simulink model "test_com_SensorFusion_SF_E10_fuerE9Daten"  (R2019b)
settings: Solver=FixedStepDiscrete  StartTime=0  StopTime=85  FixedStep=0.001  RelTol=1e-3
undefined symbols (not defined in the file or in its folder): BxTM, ByTM, CxTM, CyTM, g, gamma_stat_front, gamma_stat_rear, gearbox_ratio, l_F, l_R, m_sprung, m_unsprung_quarter, mag_calib_front_center, mag_calib_front_compmatrix, mag_calib_rear_center, mag_calib_rear_compmatrix, param, switch_VelYcalculation_pSF, testStart_VelX_pSF, testVelY_pSF, tire_r_dyn, track_angle_front, track_width_front, track_width_rear, v2o_x, wheel_kinematics_breakpoints, wheel_kinematics_FL_data, wheel_kinematics_FR_data, wheelbase, x9DFrontX, x9DFrontY, x9DRearX, x9DRearY
libraries: SignalProcessingSensorFusionLib x30, simulink x3
(part 1 of 7)
settings Model: DataDictionary=dd_SensorFusion.sldd  EnableAccessToBaseWorkspace=off  SnapshotInterval=100  Creator=daniel  LastModifiedBy=laura
settings DataIOCC: ExternalInput=VD_Gyro_Front_Accel_X, VD_Gyro_Front_Accel_Y, VD_Gyro_Front_Accel_Z,VD_Gyro_Front_ARate_X, VD_Gyro_Front_ARate_Y, VD_Gyro_Front_ARate_Z, VD_Gyro_Front_Comp_X, VD_Gyro_Front_Comp_Y, VD_Gyro_Front_Comp_Z, VD_Gyro_Front_Temp, VD_Gyro_Rear_Accel_X, VD_Gyro_Rear_Accel_Y, VD_Gyro_Rear_Accel_Z, VD_Gyro_Rear_ARate_X, VD_Gyro_Rear_ARate_Y, VD_Gyro_Rear_ARate_Z, VD_Gyro_Rear_Comp_X, VD_Gyro_Rear_Comp_Y, VD_Gyro_Rear_Comp_Z, VD_Gyro_Rear_Temp, VD_V2O_SpeedLongitudinal, VD_V2O_SpeedLateral, PT_MotorSpeed_FL, PT_MotorSpeed_FR, PT_MotorSpeed_RL, PT_MotorSpeed_RR, VD_Suspension_Hall_FL, VD_Suspension_Hall_FR, VD_Suspension_Hall_RL, VD_Suspension_Hall_RR, VD_SteeringWheelAngle  LimitDataPoints=on  LoadExternalInput=on  SaveFormat=Array  SaveOutput=off  SignalLogging=off  DSMLogging=off  SaveTime=off  ReturnWorkspaceOutputs=off
settings OptimizationCC: DefaultParameterBehavior=Inlined  UseDivisionForNetSlopeComputation=on  StateBitsets=on  DataBitsets=on  LifeSpan=1  EfficientTunableParamExpr=on
settings DebuggingCC: SolverPrmCheckMsg=warning  ParameterPrecisionLossMsg=none  AllowSymbolicDim=off  SFUnexpectedBacktrackingDiag=warning  SFNoUnconditionalDefaultTransitionDiag=warning  SFExecutionAtInitializationDiag=none  ArithmeticOperatorsInVariantConditions=warning
settings HardwareCC: ProdBitPerPointer=32  ProdBitPerSizeT=32  ProdBitPerPtrDiffT=32  ProdLargestAtomicInteger=Long  ProdLargestAtomicFloat=Double  ProdEndianess=BigEndian  ProdWordSize=32  ProdHWDeviceType=Texas Instruments->TMS570 Cortex-R4
settings ModelReferenceCC: PropagateSignalLabelsOutOfModel=off
settings SFSimCC: SimUseLocalCustomCode=off  SimBuildMode=sf_nonincremental_build  MATLABDynamicMemAlloc=off  CustomCodeUndefinedFunction=UseInterfaceOnly
settings RTWCC: SystemTargetFile=ert.tlc  GenCodeOnly=on  TemplateMakefile=ert_default_tmf  GenerateReport=on  RTWUseLocalCustomCode=off  BuildConfiguration=Faster Runs  IncludeHyperlinkInReport=on  LaunchReport=on  GenerateTraceReport=on
settings CodeAppCC: IgnoreCustomStorageClasses=off  SFDataObjDesc=on  StateflowObjectComments=on
settings ERTTargetCC: MultiwordLength=2048  GenerateSampleERTMain=on  InlinedParameterPlacement=NonHierarchical  ERTCustomFileTemplate=example_file_process.tlc  ConvertIfToSwitch=off  SuppressUnreachableDefaultCases=off
settings ConfigComp: CovMetricSettings=dw  CovHtmlReporting=on  CovSaveCumulativeToWorkspaceVar=on  CovSaveSingleToWorkspaceVar=on  CovExternalEMLEnable=off  CovSFcnEnable=off
settings SimscapeCC: SimscapeNormalizeSystem=off
settings ConfigurationSet: Description=SimMechanics 2G

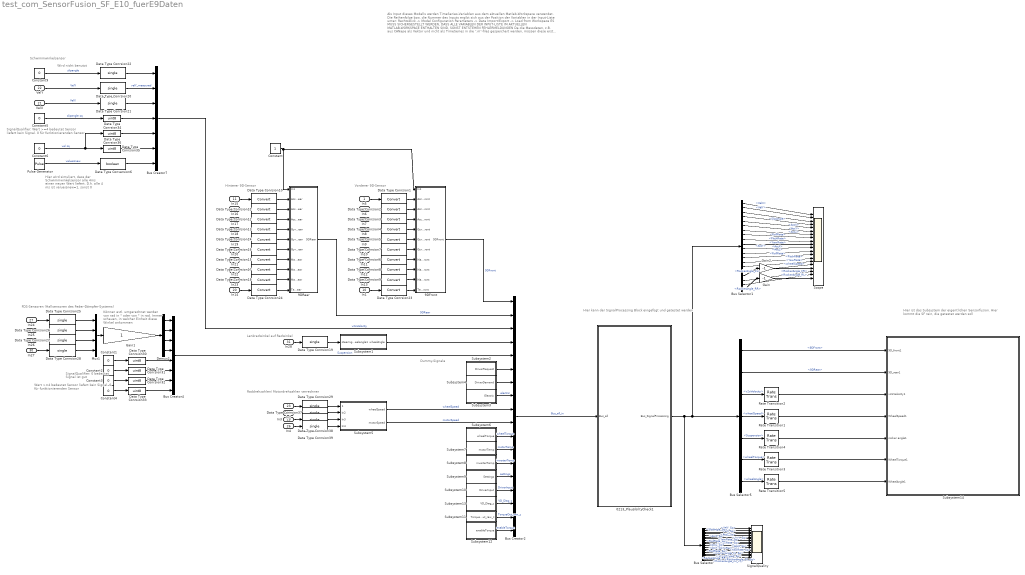
== system test_com_SensorFusion_SF_E10_fuerE9Daten ==
  note: Als Input dieses Modells werden TimeSeries-Variablen aus dem aktuellen Matlab-Workspace verwendet.
      | Die Reihenfolge bzw. die Nummer des Inputs ergibt sich aus der Position der Variablen in der Input-Liste unter:
      | Rechtsklick -> Model Configuration Parameters -> Data Import/Export -> Load from Workspace
      |
      | ES MUSS SICHERGESTELLT WERDEN, DASS ALLE VARIABLEN DER INPUT-LISTE IM AKTUELLEN
      | MATLAB-WORKSPACE ENTHALTEN SIND, SONST ENTSTEHEN FEHLERMELDUNGEN
      |
      | Da die Messdaten, z.B. aus CANape als Vektor und nicht als TimeSeries in die ".m"-files gespeichert werden,
      | müssen diese erst konvertiert werden. Es gibt unterschiedliche Matlab-Skripte mit der Benennung "LoadDataForSil",
      | die aus unterschiedlichen Messdaten, die als ".m"-files vorhanden sind, TimeSeries zu erstellen.
  note: Hier kann der SignalProcessing Block eingefügt und getestet werden
  note: Dummy-Signale
  note: Lenkradwinkel auf Radwinkel
  note: Raddrehzahlen/ Motordrehzahlen verrechnen
  note: SignalQualifier:
      | 0 bedeutet Signal ist gut
  note: Können evtl. umgerechnet werden
      | von rad in ° oder von ° in rad.
      | Immer schauen, in welcher Einheit
      | diese Winkel ankommen
  note: FDS-Sensoren (Hallsensoren des Feder-Dämpfer-Systems)
  note: Schwimmwinkelsensor
  note: Hier wird simuliert,
      | dass der Schwimmwinkelsensor
      | alle 4ms einen neuen Wert liefert.
      | D.h. alle 4 ms ist valueisnew=1,
      | sonst 0
  note: Wird nicht benutzt
  note: Hinterer 9D-Sensor
  note: Vorderer 9D-Sensor
  note: Hier ist das Subsystem der eigentlichen Sensorfusion.
      | Hier kommt die SF rein, die getestet werden soll
  note: Wert >=4 bedeutet Sensor liefert kein Signal.
      |  0 für funktionierenden Sensor
  note: SignalQualifier:
      | Wert >=4 bedeutet Sensor liefert kein Signal.
      |  0 für funktionierenden Sensor
  In5 : Inport  OutDataTypeStr=single  LockScale=on
  In6 : Inport  Port=2
  In7 : Inport  Port=3
  In8 : Inport  Port=4
  In9 : Inport  Port=5
  In10 : Inport  Port=6
  In11 : Inport  Port=7
  In12 : Inport  Port=8
  In13 : Inport  Port=9
  In1 : Inport  Port=10
  In15 : Inport  Port=11
  In16 : Inport  Port=12
  In17 : Inport  Port=13
  In18 : Inport  Port=14
  In19 : Inport  Port=15
  In20 : Inport  Port=16
  In21 : Inport  Port=17
  In22 : Inport  Port=18
  In23 : Inport  Port=19
  In14 : Inport  Port=20
  VelX : Inport  Port=21
  VelY : Inport  Port=22
  " " : Inport  Port=23
  In2 : Inport  Port=24
  In3 : Inport  Port=25
  In4 : Inport  Port=26
  In24 : Inport  Port=27
  In25 : Inport  Port=28
  In26 : Inport  Port=29
  In27 : Inport  Port=30
  In28 : Inport  Port=31
  0213_PlausibiltyCheck1 : Subsystem
  9DFront : Subsystem
  9DRear : Subsystem
  Bus Creator2 : BusCreator  Inputs=18
  Bus Creator4 : BusCreator  Inputs=8  OutDataTypeStr=Bus: control_Suspension
      settings: InheritFromInputs=off
  Bus Creator7 : BusCreator  Inputs=7  OutDataTypeStr=Bus: control_Velocity
      settings: InheritFromInputs=off
  Bus Selector : BusSelector  OutputSignals=v2oVelocity.VelX_Sq,v2oVelocity.VelY_Sq,v2oVelocity.SlipAngle_Sq,9DFront.AccX_Sq,9DFront.AccY_Sq,9DFront.AccZ_Sq,9DFront.RollRate_Sq,9DFront.PitchRate_Sq,9DFront.YawRate_Sq,9DRear.AccX_Sq,9DRear.AccY_Sq,9DRear.AccZ_Sq,9DRear.RollRate_Sq,9DRear.PitchRate_Sq,9DRear.YawRate_Sq,wheelSpeed_Sq,Suspension.RockerAngle_FL_Sq,Suspension.RockerAngle_FR_Sq,Suspension.RockerAngle_RL_Sq,Suspension.RockerAngle_RR_Sq
  Bus Selector1 : BusSelector  OutputSignals=v2oVelocity.VelX,v2oVelocity.VelY,v2oVelocity.SlipAngle,9DFront.AccX,9DFront.AccY,9DFront.AccZ,9DFront.RollRate,9DFront.PitchRate,9DFront.YawRate,9DRear.AccX,9DRear.AccY,9DRear.AccZ,9DRear.RollRate,9DRear.PitchRate,9DRear.YawRate,wheelSpeed,Suspension.RockerAngle_FL,Suspension.RockerAngle_FR,Suspension.RockerAngle_RL,Suspension.RockerAngle_RR
  Bus Selector5 : BusSelector  OutputSignals=9DFront,9DRear,v2oVelocity,wheelSpeed,Suspension,wheelTorque,wheelAngle
  Constant : Constant  OutDataTypeStr=single
  Constant{1..6} (6 alike) : Constant  Value=0
  Constant9 : Constant  Value=0  OutDataTypeStr=Inherit: Inherit via back propagation
  Data Type Conrsion{1..18,23..24} (20 alike) : DataTypeConversion
  Data Type Conrsion{19..22,25..29,37..39} (12 alike) : DataTypeConversion  OutDataTypeStr=single
  Data Type Conrsion{30..36} (7 alike) : DataTypeConversion  OutDataTypeStr=uint8
  Data Type Conversion6 : DataTypeConversion  OutDataTypeStr=boolean
  Demux2 : Demux
  Gain : Gain  Gain=-1
  Gain1 : Gain
  Gain2 : Gain  Gain=-1
  Mux1 : Mux
  Pulse Generator : DiscretePulseGenerator  Period=4  SampleTime=0.001  VectorParams1D=off
  Rate Transition{1..5} (5 alike) : RateTransition  Deterministic=off  OutPortSampleTime=0.002
  Scope : Scope  NumInputPorts=20
  SignalQuality : Scope  NumInputPorts=20
  Subsystem1 : Subsystem
  Subsystem10 : Subsystem
  Subsystem11 : Subsystem
  Subsystem12 : Subsystem
  Subsystem13 : Subsystem
  Subsystem14 : Subsystem
  Subsystem2 : Subsystem
  Subsystem3 : Subsystem
  Subsystem4 : Subsystem
  Subsystem5 : Subsystem
  Subsystem6 : Subsystem
  Subsystem7 : Subsystem
  Subsystem8 : Subsystem
  Subsystem9 : Subsystem
  wires:
  In5/1 -> Data Type Conrsion1/1
  In6/1 -> Data Type Conrsion2/1
  In7/1 -> Data Type Conrsion3/1
  In8/1 -> Data Type Conrsion4/1
  In9/1 -> Data Type Conrsion5/1
  In10/1 -> Data Type Conrsion7/1
  In11/1 -> Data Type Conrsion6/1
  In12/1 -> Data Type Conrsion8/1
  In13/1 -> Data Type Conrsion9/1
  Data Type Conrsion23/1 -> 9DFront/11(Temp9DFront)
  Data Type Conrsion1/1 -> 9DFront/2(AccXFront)
  Data Type Conrsion2/1 -> 9DFront/3(AccYFront)
  Data Type Conrsion3/1 -> 9DFront/4(AccZFront)
  Data Type Conrsion4/1 -> 9DFront/5(GyroXFront)
  Data Type Conrsion5/1 -> 9DFront/6(GyroYFront)
  Data Type Conrsion7/1 -> 9DFront/7(GyroZFront)
  Data Type Conrsion6/1 -> 9DFront/8(MagXFront)
  Data Type Conrsion8/1 -> 9DFront/9(MagYFront)
  Data Type Conrsion9/1 -> 9DFront/10(MagZFront)
  In22/1 -> Data Type Conrsion17/1
  In21/1 -> Data Type Conrsion15/1
  In20/1 -> Data Type Conrsion16/1
  In19/1 -> Data Type Conrsion14/1
  In18/1 -> Data Type Conrsion13/1
  In17/1 -> Data Type Conrsion12/1
  In16/1 -> Data Type Conrsion11/1
  In15/1 -> Data Type Conrsion10/1
  In23/1 -> Data Type Conrsion18/1
  Data Type Conrsion10/1 -> 9DRear/2(AccXRear)
  Data Type Conrsion11/1 -> 9DRear/3(AccYRear)
  Data Type Conrsion12/1 -> 9DRear/4(AccZRear)
  Data Type Conrsion13/1 -> 9DRear/5(GyroXRear)
  Data Type Conrsion14/1 -> 9DRear/6(GyroYRear)
  Data Type Conrsion16/1 -> 9DRear/7(GyroZRear)
  Data Type Conrsion15/1 -> 9DRear/8(MagXRear)
  Data Type Conrsion17/1 -> 9DRear/9(MagYRear)
  Data Type Conrsion18/1 -> 9DRear/10(MagZRear)
  In1/1 -> Data Type Conrsion23/1
  In14/1 -> Data Type Conrsion24/1
  Data Type Conrsion24/1 -> 9DRear/11(Temp9DRear)
  In27/1 -> Data Type Conrsion28/1
  In26/1 -> Data Type Conrsion27/1
  In25/1 -> Data Type Conrsion26/1
  Data Type Conrsion26/1 -> Mux1/2
  In24/1 -> Data Type Conrsion25/1
  Data Type Conrsion28/1 -> Mux1/4
  Data Type Conrsion25/1 -> Mux1/1
  Data Type Conrsion27/1 -> Mux1/3
  Gain1/1 -> Demux2/1
  Mux1/1 -> Gain1/1
  Demux2/1 -> Bus Creator4/1
  Demux2/2 -> Bus Creator4/2
  Demux2/3 -> Bus Creator4/3
  Demux2/4 -> Bus Creator4/4
  Constant1/1 -> Data Type Conrsion30/1
  Constant2/1 -> Data Type Conrsion31/1
  Constant3/1 -> Data Type Conrsion32/1
  Constant4/1 -> Data Type Conrsion33/1
  Data Type Conrsion30/1 -> Bus Creator4/5
  Data Type Conrsion31/1 -> Bus Creator4/6
  Data Type Conrsion32/1 -> Bus Creator4/7
  Data Type Conrsion33/1 -> Bus Creator4/8
  VelY/1 -> Data Type Conrsion20/1  "VelY"
  Data Type Conrsion20/1 -> Bus Creator7/2  "velY_measured"
  Data Type Conrsion21/1 -> Bus Creator7/3
  Constant9/1 -> Data Type Conrsion22/1  "slipangle"
  Data Type Conrsion22/1 -> Bus Creator7/1
  VelX/1 -> Data Type Conrsion21/1  "VelX"
  Pulse Generator/1 -> Data Type Conversion6/1  "valueisnew"
  Data Type Conversion6/1 -> Bus Creator7/7
  Constant6/1 -> Data Type Conrsion36/1, Data Type Conrsion35/1  "vel sq"
  Data Type Conrsion35/1 -> Bus Creator7/6
  Constant5/1 -> Data Type Conrsion34/1  "slipangle sq"
  Data Type Conrsion36/1 -> Bus Creator7/5
  Data Type Conrsion34/1 -> Bus Creator7/4
  Subsystem10/1(DriverInput) -> Bus Creator2/15  "DriverInput"
  Bus Creator2/1 -> 0213_PlausibiltyCheck1/1(Bus_all)  "Bus_all_in"
  Subsystem8/1(inverterTemp) -> Bus Creator2/13  "inverterTemp"
  Subsystem6/1(wheelTorque) -> Bus Creator2/11  "wheelTorque"
  Bus Creator7/1 -> Bus Creator2/3  "v2oVelocity"
  Subsystem12/1(enableTorque) -> Bus Creator2/18  "enableTorque"
  Subsystem7/1(motorTemp) -> Bus Creator2/12  "motorTemp"
  9DRear/1(9DRear) -> Bus Creator2/2  "9DRear"
  Subsystem9/1(Settings) -> Bus Creator2/14  "settings"
  Subsystem3/1(Electric) -> Bus Creator2/8  "electric"
  Bus Creator4/1 -> Bus Creator2/5  "Suspension"
  Subsystem11/1(TorqueOut_raw_z) -> Bus Creator2/17  "TorqueOut_raw_z"
  9DFront/1(9DFront) -> Bus Creator2/1  "9DFront"
  Subsystem1/1("wheelAngle ") -> Bus Creator2/4
  Subsystem2/1(DriverRequest) -> Bus Creator2/6
  Subsystem4/1(DriverDemand) -> Bus Creator2/7
  " "/1 -> Data Type Conrsion29/1
  In2/1 -> Data Type Conrsion37/1
  In3/1 -> Data Type Conrsion38/1
  In4/1 -> Data Type Conrsion39/1
  Subsystem5/1(wheelSpeed) -> Bus Creator2/9  "wheelSpeed"
  Subsystem5/2(motorSpeed) -> Bus Creator2/10  "motorSpeed"
  Subsystem13/1(VD_Diag_z) -> Bus Creator2/16  "VD_Diag_z"
  Bus Selector5/5 -> Rate Transition4/1  "<Suspension>"
  Rate Transition1/1 -> Subsystem14/4(WheelSpeed1)
  Bus Selector5/1 -> Subsystem14/1(9D_front1)  "<9DFront>"
  Rate Transition5/1 -> Subsystem14/7(WheelAngle1)
  Bus Selector5/6 -> Rate Transition3/1  "<wheelTorque>"
  Rate Transition4/1 -> Subsystem14/5(rocker angle1)
  Bus Selector5/3 -> Rate Transition2/1  "<v2oVelocity>"
  Bus Selector5/2 -> Subsystem14/2(9D_rear1)  "<9DRear>"
  Bus Selector5/4 -> Rate Transition1/1  "<wheelSpeed>"
  Bus Selector5/7 -> Rate Transition5/1  "<wheelAngle>"
  Rate Transition3/1 -> Subsystem14/6(WheelTorque1)
  Rate Transition2/1 -> Subsystem14/3(v2oVelocity1)
  0213_PlausibiltyCheck1/1(Bus_SignalProcessing) -> Bus Selector/1, Bus Selector1/1, Bus Selector5/1
  In28/1 -> Data Type Conrsion19/1
  Data Type Conrsion19/1 -> Subsystem1/1(steeringwheelangle1)
  Data Type Conrsion29/1 -> Subsystem5/1(" ")
  Data Type Conrsion37/1 -> Subsystem5/2(In2)
  Data Type Conrsion38/1 -> Subsystem5/3(In3)
  Data Type Conrsion39/1 -> Subsystem5/4(In4)
  Gain2/1 -> Scope/17
  Bus Selector1/9 -> Scope/9  "<YawRate>"
  Bus Selector1/17 -> Gain2/1  "<RockerAngle_FL>"
  Bus Selector1/1 -> Scope/1  "<VelX>"
  Bus Selector1/13 -> Scope/13  "<RollRate>"
  Bus Selector1/11 -> Scope/11  "<AccY>"
  Bus Selector1/15 -> Scope/15  "<YawRate>"
  Gain/1 -> Scope/20
  Bus Selector1/5 -> Scope/5  "<AccY>"
  Bus Selector1/10 -> Scope/10  "<AccX>"
  Bus Selector1/14 -> Scope/14  "<PitchRate>"
  Bus Selector1/4 -> Scope/4  "<AccX>"
  Bus Selector1/16 -> Scope/16  "<wheelSpeed>"
  Bus Selector1/19 -> Scope/19  "<RockerAngle_RL>"
  Bus Selector1/20 -> Gain/1  "<RockerAngle_RR>"
  Bus Selector1/8 -> Scope/8  "<PitchRate>"
  Bus Selector1/7 -> Scope/7  "<RollRate>"
  Bus Selector1/12 -> Scope/12  "<AccZ>"
  Bus Selector1/6 -> Scope/6  "<AccZ>"
  Bus Selector1/18 -> Scope/18  "<RockerAngle_FR>"
  Bus Selector1/2 -> Scope/2  "<VelY>"
  Bus Selector1/3 -> Scope/3  "<SlipAngle>"
  Bus Selector/17 -> SignalQuality/17  "<RockerAngle_FL_Sq>"
  Bus Selector/2 -> SignalQuality/2  "<VelY_Sq>"
  Bus Selector/14 -> SignalQuality/14  "<PitchRate_Sq>"
  Bus Selector/1 -> SignalQuality/1  "<VelX_Sq>"
  Bus Selector/16 -> SignalQuality/16  "<wheelSpeed_Sq>"
  Bus Selector/6 -> SignalQuality/6  "<AccZ_Sq>"
  Bus Selector/4 -> SignalQuality/4  "<AccX_Sq>"
  Bus Selector/5 -> SignalQuality/5  "<AccY_Sq>"
  Bus Selector/8 -> SignalQuality/8  "<PitchRate_Sq>"
  Bus Selector/19 -> SignalQuality/19  "<RockerAngle_RL_Sq>"
  Bus Selector/12 -> SignalQuality/12  "<AccZ_Sq>"
  Bus Selector/7 -> SignalQuality/7  "<RollRate_Sq>"
  Bus Selector/10 -> SignalQuality/10  "<AccX_Sq>"
  Bus Selector/20 -> SignalQuality/20  "<RockerAngle_RR_Sq>"
  Bus Selector/9 -> SignalQuality/9  "<YawRate_Sq>"
  Bus Selector/13 -> SignalQuality/13  "<RollRate_Sq>"
  Bus Selector/3 -> SignalQuality/3  "<SlipAngle_Sq>"
  Bus Selector/11 -> SignalQuality/11  "<AccY_Sq>"
  Bus Selector/15 -> SignalQuality/15  "<YawRate_Sq>"
  Bus Selector/18 -> SignalQuality/18  "<RockerAngle_FR_Sq>"
  Constant/1 -> 9DFront/1(In1), 9DRear/1(In1)

== system test_com_SensorFusion_SF_E10_fuerE9Daten/0213_PlausibiltyCheck1 ==
  Bus_all : Inport
  9DFront_Plausibility : Subsystem
  9DRear_Plausibility : Subsystem
  Bus Creator1 : BusCreator  Inputs=18
  Bus Selector1 : BusSelector  OutputSignals=9DFront,9DRear,v2oVelocity,wheelSpeed,Suspension,electric,wheelTorque,wheelAngle,settings,DriverInput,motorTemp,inverterTemp,motorSpeed,DriverRequest,DriverDemand,TorqueOut_raw_z,VD_Diag_z
  DriverRequest_Plausibility : Subsystem
  Suspension_Plausibility : Subsystem
  Suspension_Plausibility1 : Subsystem
  Terminator2 : Terminator
  motorSpeed_Plausibility : Subsystem
  v2oVelocity_Plausibility : Subsystem
  wheelSpeed_Plausibility : Subsystem
  Bus_SignalProcessing : Outport  VectorParamsAs1DForOutWhenUnconnected=off
  wires:
  Bus Selector1/4 -> wheelSpeed_Plausibility/1(In)  "<wheelSpeed>"
  Bus Selector1/3 -> v2oVelocity_Plausibility/1(In)  "<v2oVelocity>"
  Bus_all/1 -> Bus Selector1/1
  Bus Selector1/7 -> Bus Creator1/8  "<wheelTorque>"
  Bus Creator1/1 -> Bus_SignalProcessing/1  "Bus_all"
  Bus Selector1/2 -> 9DRear_Plausibility/1(In)  "<9DRear>"
  Bus Selector1/5 -> Suspension_Plausibility/1(In)  "<Suspension>"
  Bus Selector1/6 -> Suspension_Plausibility1/1(In)  "<electric>"
  Bus Selector1/15 -> Bus Creator1/16  "<DriverDemand>"
  Bus Selector1/16 -> Bus Creator1/17  "<TorqueOut_raw_z>"
  Bus Selector1/17 -> Bus Creator1/18  "<VD_Diag_z>"
  Bus Selector1/8 -> Bus Creator1/9  "<wheelAngle>"
  Bus Selector1/9 -> Bus Creator1/10  "<settings>"
  Bus Selector1/10 -> Bus Creator1/11  "<DriverInput>"
  Bus Selector1/11 -> Bus Creator1/12  "<motorTemp>"
  Bus Selector1/13 -> motorSpeed_Plausibility/1(In)  "<motorSpeed>"
  Bus Selector1/14 -> DriverRequest_Plausibility/1(In)  "<DriverRequest>"
  Bus Selector1/1 -> 9DFront_Plausibility/1(In)  "<9DFront>"
  9DFront_Plausibility/1(Out) -> Bus Creator1/1  "9DFront"
  9DRear_Plausibility/1(Out) -> Bus Creator1/2  "9DRear"
  v2oVelocity_Plausibility/1(Out) -> Bus Creator1/3  "v2oVelocity"
  wheelSpeed_Plausibility/1(WheelSpeed) -> Bus Creator1/4  "wheelSpeed"
  Suspension_Plausibility/1(Out) -> Bus Creator1/6  "Suspension"
  motorSpeed_Plausibility/1(WheelSpeed) -> Bus Creator1/14  "motorSpeed"
  Bus Selector1/12 -> Bus Creator1/13  "<inverterTemp>"
  DriverRequest_Plausibility/1(Out) -> Bus Creator1/15  "DriverRequest"
  Suspension_Plausibility1/1(Out) -> Bus Creator1/7  "electric"
  wheelSpeed_Plausibility/2(WheelSpeed_Sq) -> Bus Creator1/5  "wheelSpeed_Sq"
  motorSpeed_Plausibility/2(WheelSpeed_Sq) -> Terminator2/1

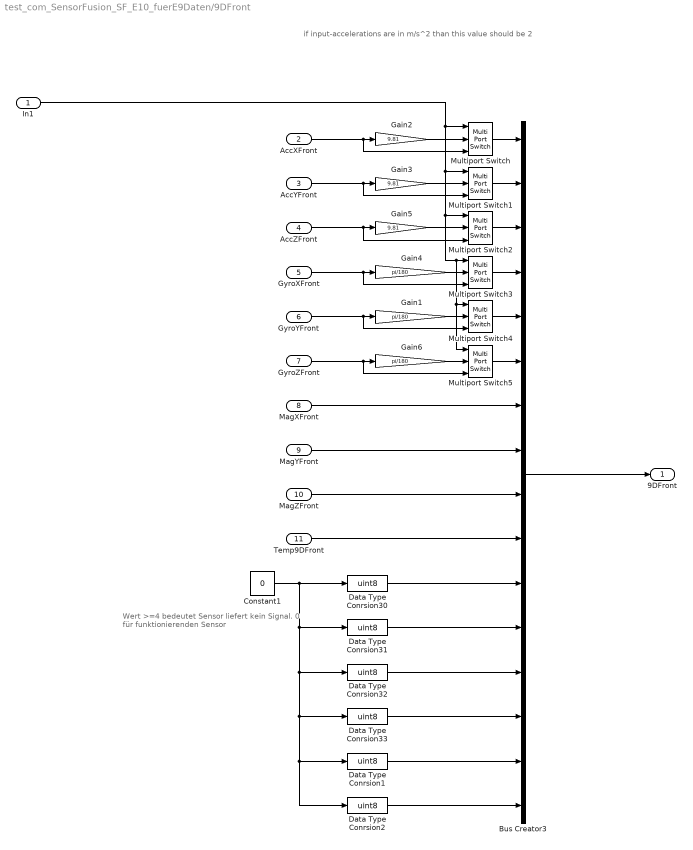
== system test_com_SensorFusion_SF_E10_fuerE9Daten/9DFront ==
  note: if input-accelerations are in m/s^2 than this value should be 2
  note: Wert >=4 bedeutet Sensor liefert kein Signal.
      |  0 für funktionierenden Sensor
  In1 : Inport
  AccXFront : Inport  Port=2
  AccYFront : Inport  Port=3
  AccZFront : Inport  Port=4
  GyroXFront : Inport  Port=5
  GyroYFront : Inport  Port=6
  GyroZFront : Inport  Port=7
  MagXFront : Inport  Port=8
  MagYFront : Inport  Port=9
  MagZFront : Inport  Port=10
  Temp9DFront : Inport  Port=11
  Bus Creator3 : BusCreator  Inputs=16  OutDataTypeStr=Bus: control_9D
      settings: InheritFromInputs=off
  Constant1 : Constant  Value=0
  Data Type Conrsion{1..2,30..33} (6 alike) : DataTypeConversion  OutDataTypeStr=uint8
  Gain1 : Gain  Gain=pi/180
  Gain2 : Gain  Gain=9.81
  Gain3 : Gain  Gain=9.81
  Gain4 : Gain  Gain=pi/180
  Gain5 : Gain  Gain=9.81
  Gain6 : Gain  Gain=pi/180
  Multiport Switch{,1..5} (6 alike) : MultiPortSwitch  Inputs=2
  9DFront : Outport  OutDataTypeStr=Bus: control_9D  VectorParamsAs1DForOutWhenUnconnected=off
  wires:
  AccXFront/1 -> Multiport Switch/3, Gain2/1
  Temp9DFront/1 -> Bus Creator3/10
  MagZFront/1 -> Bus Creator3/9
  Gain2/1 -> Multiport Switch/2
  Bus Creator3/1 -> 9DFront/1
  MagYFront/1 -> Bus Creator3/8
  MagXFront/1 -> Bus Creator3/7
  GyroXFront/1 -> Multiport Switch3/3, Gain4/1
  Gain4/1 -> Multiport Switch3/2
  Data Type Conrsion30/1 -> Bus Creator3/11
  Data Type Conrsion31/1 -> Bus Creator3/12
  Data Type Conrsion32/1 -> Bus Creator3/13
  Data Type Conrsion33/1 -> Bus Creator3/14
  Data Type Conrsion2/1 -> Bus Creator3/16
  Data Type Conrsion1/1 -> Bus Creator3/15
  In1/1 -> Multiport Switch2/1, Multiport Switch5/1, Multiport Switch4/1, Multiport Switch3/1, Multiport Switch1/1, Multiport Switch/1
  Multiport Switch/1 -> Bus Creator3/1
  Multiport Switch1/1 -> Bus Creator3/2
  Gain3/1 -> Multiport Switch1/2
  AccYFront/1 -> Multiport Switch1/3, Gain3/1
  Multiport Switch2/1 -> Bus Creator3/3
  Gain5/1 -> Multiport Switch2/2
  AccZFront/1 -> Multiport Switch2/3, Gain5/1
  Multiport Switch3/1 -> Bus Creator3/4
  Gain1/1 -> Multiport Switch4/2
  Multiport Switch4/1 -> Bus Creator3/5
  GyroYFront/1 -> Multiport Switch4/3, Gain1/1
  Gain6/1 -> Multiport Switch5/2
  Multiport Switch5/1 -> Bus Creator3/6
  GyroZFront/1 -> Multiport Switch5/3, Gain6/1
  Constant1/1 -> Data Type Conrsion30/1, Data Type Conrsion31/1, Data Type Conrsion32/1, Data Type Conrsion33/1, Data Type Conrsion2/1, Data Type Conrsion1/1

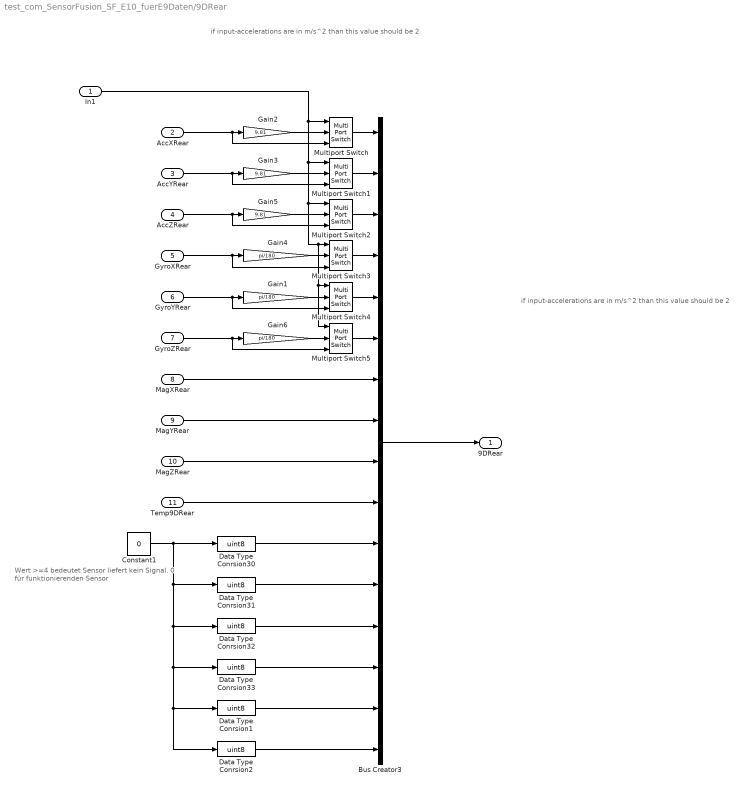
== system test_com_SensorFusion_SF_E10_fuerE9Daten/9DRear ==
  note: Wert >=4 bedeutet Sensor liefert kein Signal.
      |  0 für funktionierenden Sensor
  note: if input-accelerations are in m/s^2 than this value should be 2
  note: if input-accelerations are in m/s^2 than this value should be 2
  In1 : Inport
  AccXRear : Inport  Port=2
  AccYRear : Inport  Port=3
  AccZRear : Inport  Port=4
  GyroXRear : Inport  Port=5
  GyroYRear : Inport  Port=6
  GyroZRear : Inport  Port=7
  MagXRear : Inport  Port=8
  MagYRear : Inport  Port=9
  MagZRear : Inport  Port=10
  Temp9DRear : Inport  Port=11
  Bus Creator3 : BusCreator  Inputs=16  OutDataTypeStr=Bus: control_9D
      settings: InheritFromInputs=off
  Constant1 : Constant  Value=0
  Data Type Conrsion{1..2,30..33} (6 alike) : DataTypeConversion  OutDataTypeStr=uint8
  Gain1 : Gain  Gain=pi/180
  Gain2 : Gain  Gain=9.81
  Gain3 : Gain  Gain=9.81
  Gain4 : Gain  Gain=pi/180
  Gain5 : Gain  Gain=9.81
  Gain6 : Gain  Gain=pi/180
  Multiport Switch{,1..5} (6 alike) : MultiPortSwitch  Inputs=2
  9DRear : Outport  OutDataTypeStr=Bus: control_9D  VectorParamsAs1DForOutWhenUnconnected=off
  wires:
  Bus Creator3/1 -> 9DRear/1
  Temp9DRear/1 -> Bus Creator3/10
  MagXRear/1 -> Bus Creator3/7
  MagZRear/1 -> Bus Creator3/9
  MagYRear/1 -> Bus Creator3/8
  Constant1/1 -> Data Type Conrsion2/1, Data Type Conrsion1/1, Data Type Conrsion33/1, Data Type Conrsion32/1, Data Type Conrsion31/1, Data Type Conrsion30/1
  Data Type Conrsion31/1 -> Bus Creator3/12
  Data Type Conrsion2/1 -> Bus Creator3/16
  Data Type Conrsion32/1 -> Bus Creator3/13
  Data Type Conrsion33/1 -> Bus Creator3/14
  Data Type Conrsion30/1 -> Bus Creator3/11
  Data Type Conrsion1/1 -> Bus Creator3/15
  Multiport Switch1/1 -> Bus Creator3/2
  GyroYRear/1 -> Multiport Switch4/3, Gain1/1
  AccYRear/1 -> Multiport Switch1/3, Gain3/1
  Multiport Switch5/1 -> Bus Creator3/6
  Gain6/1 -> Multiport Switch5/2
  Gain5/1 -> Multiport Switch2/2
  Multiport Switch/1 -> Bus Creator3/1
  In1/1 -> Multiport Switch2/1, Multiport Switch5/1, Multiport Switch4/1, Multiport Switch3/1, Multiport Switch1/1, Multiport Switch/1
  Multiport Switch3/1 -> Bus Creator3/4
  Gain2/1 -> Multiport Switch/2
  AccZRear/1 -> Multiport Switch2/3, Gain5/1
  Multiport Switch4/1 -> Bus Creator3/5
  GyroXRear/1 -> Multiport Switch3/3, Gain4/1
  AccXRear/1 -> Multiport Switch/3, Gain2/1
  GyroZRear/1 -> Multiport Switch5/3, Gain6/1
  Gain1/1 -> Multiport Switch4/2
  Gain3/1 -> Multiport Switch1/2
  Multiport Switch2/1 -> Bus Creator3/3
  Gain4/1 -> Multiport Switch3/2

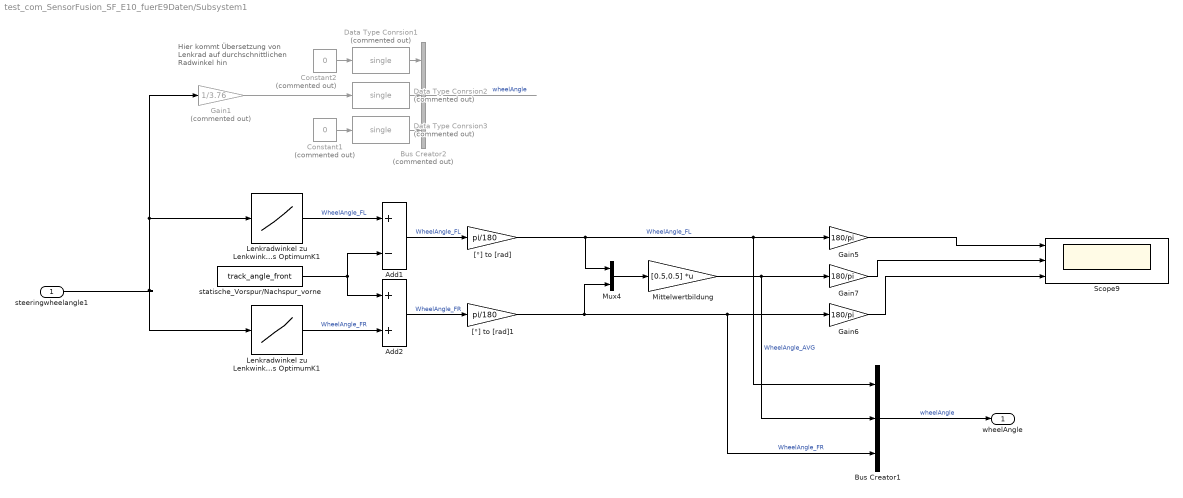
== system test_com_SensorFusion_SF_E10_fuerE9Daten/Subsystem1 ==
  note: Hier kommt Übersetzung
      | von Lenkrad auf
      | durchschnittlichen
      | Radwinkel hin
  steeringwheelangle1 : Inport
  Add1 : Sum  Inputs=+-
  Add2 : Sum
  Bus Creator1 : BusCreator  Inputs=3
  Bus Creator2 : BusCreator  Commented=on  Inputs=3  OutDataTypeStr=Bus: control_WheelAngle
      settings: InheritFromInputs=off
  Constant1 : Constant  Commented=on  Value=0
  Constant2 : Constant  Commented=on  Value=0
  Data Type Conrsion1 : DataTypeConversion  Commented=on  OutDataTypeStr=single
  Data Type Conrsion2 : DataTypeConversion  Commented=on  OutDataTypeStr=single
  Data Type Conrsion3 : DataTypeConversion  Commented=on  OutDataTypeStr=single
  Gain1 : Gain  Commented=on  Gain=1/3.76
  Gain5 : Gain  Gain=180/pi
  Gain6 : Gain  Gain=180/pi
  Gain7 : Gain  Gain=180/pi
  Lenkradwinkel zu Lenkwinkel_vl aus OptimumK1 : Lookup_n-D  NumberOfTableDimensions=1  BreakpointsForDimension1=wheel_kinematics_breakpoints  Table=wheel_kinematics_FL_data  InternalRulePriority=Speed  RndMeth=Simplest  InputSameDT=on
  Lenkradwinkel zu Lenkwinkel_vr aus OptimumK1 : Lookup_n-D  NumberOfTableDimensions=1  BreakpointsForDimension1=wheel_kinematics_breakpoints  Table=wheel_kinematics_FR_data  InternalRulePriority=Speed  RndMeth=Simplest  InputSameDT=on
  Mittelwertbildung : Gain  Gain=[0.5,0.5]  Multiplication=Matrix(K*u)
  Mux4 : Mux  Inputs=2
  Scope9 : Scope  NumInputPorts=3
  "[°] to [rad]" : Gain  Gain=pi/180
  "[°] to [rad]1" : Gain  Gain=pi/180
  statische_Vorspur/Nachspur_vorne : Constant  Value=track_angle_front
  "wheelAngle " : Outport  VectorParamsAs1DForOutWhenUnconnected=off
  wires:
  Gain5/1 -> Scope9/1
  Add2/1 -> "[°] to [rad]1"/1  "WheelAngle_FR"
  Data Type Conrsion2/1 -> Bus Creator2/2
  Data Type Conrsion3/1 -> Bus Creator2/3
  Mittelwertbildung/1 -> Bus Creator1/2, Gain7/1  "WheelAngle_AVG"
  Gain7/1 -> Scope9/2
  Bus Creator1/1 -> "wheelAngle "/1  "wheelAngle"
  Mux4/1 -> Mittelwertbildung/1
  Gain6/1 -> Scope9/3
  steeringwheelangle1/1 -> Gain1/1, Lenkradwinkel zu Lenkwinkel_vl aus OptimumK1/1, Lenkradwinkel zu Lenkwinkel_vr aus OptimumK1/1
  Constant2/1 -> Data Type Conrsion1/1
  Add1/1 -> "[°] to [rad]"/1  "WheelAngle_FL"
  Lenkradwinkel zu Lenkwinkel_vl aus OptimumK1/1 -> Add1/1  "WheelAngle_FL"
  "[°] to [rad]"/1 -> Bus Creator1/1, Gain5/1, Mux4/1  "WheelAngle_FL"
  statische_Vorspur/Nachspur_vorne/1 -> Add1/2, Add2/1
  Data Type Conrsion1/1 -> Bus Creator2/1
  Gain1/1 -> Data Type Conrsion2/1
  Constant1/1 -> Data Type Conrsion3/1
  Lenkradwinkel zu Lenkwinkel_vr aus OptimumK1/1 -> Add2/2  "WheelAngle_FR"
  Bus Creator2/1 -> ?  "wheelAngle"
  "[°] to [rad]1"/1 -> Bus Creator1/3, Gain6/1, Mux4/2  "WheelAngle_FR"

== system test_com_SensorFusion_SF_E10_fuerE9Daten/Subsystem10 ==
  Bus Creator3 : BusCreator  Inputs=9  OutDataTypeStr=Bus: control_DriverInput
      settings: InheritFromInputs=off
  Constant{1..9} (9 alike) : Constant  Value=0
  Data Type Conrsion1 : DataTypeConversion  OutDataTypeStr=uint8
  Data Type Conrsion{10..13} (4 alike) : DataTypeConversion  OutDataTypeStr=boolean
  Data Type Conrsion2 : DataTypeConversion  OutDataTypeStr=uint8
  Data Type Conrsion3 : DataTypeConversion  OutDataTypeStr=uint8
  Data Type Conrsion4 : DataTypeConversion  OutDataTypeStr=single
  Data Type Conrsion5 : DataTypeConversion  OutDataTypeStr=single
  DriverInput : Outport  OutDataTypeStr=Bus: control_DriverInput  VectorParamsAs1DForOutWhenUnconnected=off
  wires:
  Constant9/1 -> Data Type Conrsion1/1
  Constant7/1 -> Data Type Conrsion2/1
  Constant6/1 -> Data Type Conrsion3/1
  Constant5/1 -> Data Type Conrsion4/1
  Constant4/1 -> Data Type Conrsion5/1
  Constant3/1 -> Data Type Conrsion13/1
  Constant2/1 -> Data Type Conrsion12/1
  Constant1/1 -> Data Type Conrsion11/1
  Constant8/1 -> Data Type Conrsion10/1
  Bus Creator3/1 -> DriverInput/1  "DriverInput"
  Data Type Conrsion4/1 -> Bus Creator3/6
  Data Type Conrsion1/1 -> Bus Creator3/9
  Data Type Conrsion2/1 -> Bus Creator3/8
  Data Type Conrsion3/1 -> Bus Creator3/7
  Data Type Conrsion11/1 -> Bus Creator3/2
  Data Type Conrsion5/1 -> Bus Creator3/5
  Data Type Conrsion12/1 -> Bus Creator3/3
  Data Type Conrsion13/1 -> Bus Creator3/4
  Data Type Conrsion10/1 -> Bus Creator3/1

== system test_com_SensorFusion_SF_E10_fuerE9Daten/Subsystem11 ==
  Constant{,1..3} (4 alike) : Constant  Value=0
  Data Type Conrsion{1,19..22} (5 alike) : DataTypeConversion  OutDataTypeStr=single
  Mux : Mux
  TorqueOut_raw_z : Outport  VectorParamsAs1DForOutWhenUnconnected=off
  wires:
  Mux/1 -> Data Type Conrsion1/1  "TorqueOut_raw_z"
  Data Type Conrsion19/1 -> Mux/1
  Data Type Conrsion20/1 -> Mux/2
  Data Type Conrsion22/1 -> Mux/4
  Data Type Conrsion21/1 -> Mux/3
  Constant1/1 -> Data Type Conrsion20/1
  Constant/1 -> Data Type Conrsion19/1
  Constant3/1 -> Data Type Conrsion22/1
  Constant2/1 -> Data Type Conrsion21/1
  Data Type Conrsion1/1 -> TorqueOut_raw_z/1

== system test_com_SensorFusion_SF_E10_fuerE9Daten/Subsystem12 ==
  Constant{,1..3} (4 alike) : Constant  Value=0
  Data Type Conrsion{1..3,22} (4 alike) : DataTypeConversion  OutDataTypeStr=boolean
  Mux : Mux
  enableTorque : Outport  VectorParamsAs1DForOutWhenUnconnected=off
  wires:
  Constant2/1 -> Data Type Conrsion1/1
  Constant3/1 -> Data Type Conrsion22/1
  Constant/1 -> Data Type Conrsion3/1
  Constant1/1 -> Data Type Conrsion2/1
  Data Type Conrsion1/1 -> Mux/3
  Data Type Conrsion22/1 -> Mux/4
  Data Type Conrsion2/1 -> Mux/2
  Data Type Conrsion3/1 -> Mux/1
  Mux/1 -> enableTorque/1  "enableTorque"

== system test_com_SensorFusion_SF_E10_fuerE9Daten/Subsystem13 ==
  Constant8 : Constant  Value=0
  Data Type Conrsion29 : DataTypeConversion  OutDataTypeStr=uint16
  VD_Diag_z : Outport  VectorParamsAs1DForOutWhenUnconnected=off
  wires:
  Constant8/1 -> Data Type Conrsion29/1
  Data Type Conrsion29/1 -> VD_Diag_z/1  "DriverDemand"

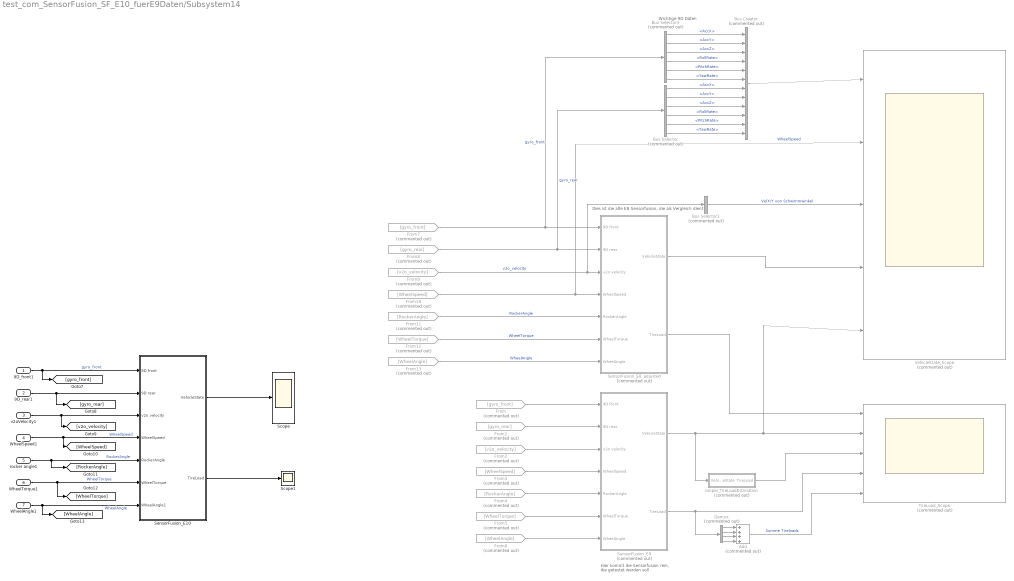
== system test_com_SensorFusion_SF_E10_fuerE9Daten/Subsystem14 ==
  note: Hier kommt die Sensorfusion rein,
      | die getestet werden soll
  note: Wichtige 9D Daten
  note: Dies ist die alte E8 Sensorfusion, die als Vergleich dient
  9D_front1 : Inport  OutDataTypeStr=Bus: control_9D  SampleTime=0.002
  9D_rear1 : Inport  Port=2  OutDataTypeStr=Bus: control_9D  SampleTime=0.002
  v2oVelocity1 : Inport  Port=3  OutDataTypeStr=Bus: control_Velocity  SampleTime=0.002
  WheelSpeed1 : Inport  Port=4  PortDimensions=4  SampleTime=0.002
  rocker angle1 : Inport  Port=5  OutDataTypeStr=Bus: control_Suspension  SampleTime=0.002
  WheelTorque1 : Inport  Port=6  PortDimensions=4  SampleTime=0.002
  WheelAngle1 : Inport  Port=7  SampleTime=0.002
  Add : Sum  Commented=on  Inputs=++++
  Bus Creator : BusCreator  Commented=on  Inputs=12
  Bus Selector : BusSelector  Commented=on  OutputSignals=AccX,AccY,AccZ,RollRate,PitchRate,YawRate
  Bus Selector1 : BusSelector  Commented=on  OutputSignals=VelY,VelX  OutputAsBus=on
  Bus Selector3 : BusSelector  Commented=on  OutputSignals=AccX,AccY,AccZ,RollRate,PitchRate,YawRate
  Demux : Demux  Commented=on
  From : From  Commented=on  GotoTag=gyro_front
  From1 : From  Commented=on  GotoTag=gyro_rear
  From10 : From  Commented=on  GotoTag=WheelSpeed
  From11 : From  Commented=on  GotoTag=RockerAngle
  From12 : From  Commented=on  GotoTag=WheelTorque
  From13 : From  Commented=on  GotoTag=WheelAngle
  From2 : From  Commented=on  GotoTag=v2o_velocity
  From3 : From  Commented=on  GotoTag=WheelSpeed
  From4 : From  Commented=on  GotoTag=RockerAngle
  From5 : From  Commented=on  GotoTag=WheelTorque
  From6 : From  Commented=on  GotoTag=WheelAngle
  From7 : From  Commented=on  GotoTag=gyro_front
  From8 : From  Commented=on  GotoTag=gyro_rear
  From9 : From  Commented=on  GotoTag=v2o_velocity
  Scope : Scope
  Scope1 : Scope
  SensorFusion_E10 : Subsystem
  SensorFusion_E8_adjusted : Subsystem  Commented=on
  SensorFusion_E9 : Subsystem  Commented=on
  TireLoad_Scope : Scope  Commented=on  NumInputPorts=5
  VehicleState_Scope : Scope  Commented=on  NumInputPorts=5
  simple_TireLoadEstimation : Subsystem  Commented=on
  wires:
  From13/1 -> SensorFusion_E8_adjusted/7(WheelAngle)  "WheelAngle"
  From/1 -> SensorFusion_E9/1(9D front)
  From12/1 -> SensorFusion_E8_adjusted/6(WheelTorque)  "WheelTorque"
  From1/1 -> SensorFusion_E9/2(9D rear)
  From8/1 -> Bus Selector/1, SensorFusion_E8_adjusted/2(9D rear)  "gyro_rear"
  From7/1 -> SensorFusion_E8_adjusted/1(9D front), Bus Selector3/1  "gyro_front"
  From6/1 -> SensorFusion_E9/7(WheelAngle)
  From2/1 -> SensorFusion_E9/3(v2o velocity)
  From11/1 -> SensorFusion_E8_adjusted/5(RockerAngle)  "RockerAngle"
  SensorFusion_E8_adjusted/2(TireLoad) -> TireLoad_Scope/1
  From5/1 -> SensorFusion_E9/6(WheelTorque)
  SensorFusion_E9/1(VehicleState) -> VehicleState_Scope/5, TireLoad_Scope/2, simple_TireLoadEstimation/1(VehicleState)
  From3/1 -> SensorFusion_E9/4(WheelSpeed)
  From10/1 -> VehicleState_Scope/2, SensorFusion_E8_adjusted/4(WheelSpeed)  "WheelSpeed"
  From9/1 -> Bus Selector1/1, SensorFusion_E8_adjusted/3(v2o velocity)  "v2o_velocity"
  From4/1 -> SensorFusion_E9/5(RockerAngle)
  SensorFusion_E9/2(TireLoad) -> TireLoad_Scope/4, Demux/1
  Bus Selector1/1 -> VehicleState_Scope/3  "VelX/Y von Schwimmwinkel"
  Bus Selector3/1 -> Bus Creator/1  "<AccX>"
  Bus Selector3/2 -> Bus Creator/2  "<AccY>"
  Bus Selector3/3 -> Bus Creator/3  "<AccZ>"
  Bus Selector3/4 -> Bus Creator/4  "<RollRate>"
  Bus Selector3/5 -> Bus Creator/5  "<PitchRate>"
  Bus Selector3/6 -> Bus Creator/6  "<YawRate>"
  Bus Selector/1 -> Bus Creator/7  "<AccX>"
  Bus Selector/2 -> Bus Creator/8  "<AccY>"
  Bus Selector/3 -> Bus Creator/9  "<AccZ>"
  Bus Selector/4 -> Bus Creator/10  "<RollRate>"
  Bus Selector/5 -> Bus Creator/11  "<PitchRate>"
  Bus Selector/6 -> Bus Creator/12  "<YawRate>"
  Bus Creator/1 -> VehicleState_Scope/1
  Demux/1 -> Add/1
  Demux/2 -> Add/2
  Demux/3 -> Add/3
  Demux/4 -> Add/4
  Add/1 -> TireLoad_Scope/5  "Summe Tireloads"
  simple_TireLoadEstimation/1(TireLoad) -> TireLoad_Scope/3
  v2oVelocity1/1 -> [v2o_velocity], SensorFusion_E10/3(v2o velocity)
  9D_rear1/1 -> [gyro_rear], SensorFusion_E10/2(9D rear)
  SensorFusion_E10/1(VehicleState) -> Scope/1
  SensorFusion_E10/2(TireLoad) -> Scope1/1
  SensorFusion_E8_adjusted/1(VehicleState) -> VehicleState_Scope/4
  9D_front1/1 -> SensorFusion_E10/1(9D front), [gyro_front]  "gyro_front"
  WheelSpeed1/1 -> [WheelSpeed], SensorFusion_E10/4(WheelSpeed)  "WheelSpeed"
  rocker angle1/1 -> SensorFusion_E10/5(RockerAngle), [RockerAngle]  "RockerAngle"
  WheelAngle1/1 -> [WheelAngle], SensorFusion_E10/7(WheelAngle1)  "WheelAngle"
  WheelTorque1/1 -> [WheelTorque], SensorFusion_E10/6(WheelTorque)  "WheelTorque"

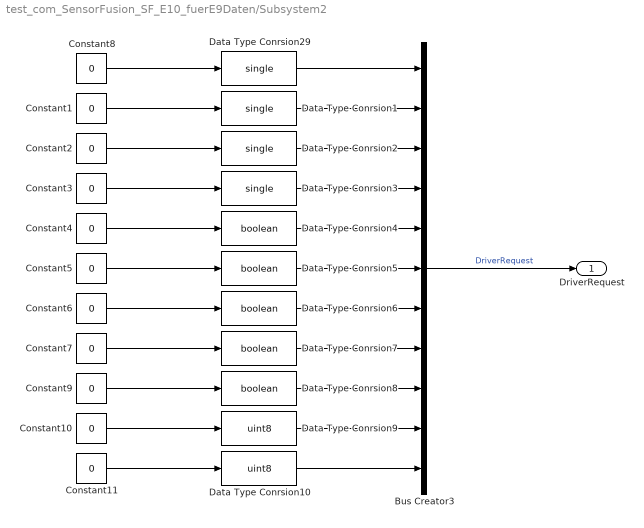
== system test_com_SensorFusion_SF_E10_fuerE9Daten/Subsystem2 ==
  Bus Creator3 : BusCreator  Inputs=11  OutDataTypeStr=Bus: control_DriverRequest
      settings: InheritFromInputs=off
  Constant{1..11} (11 alike) : Constant  Value=0
  Data Type Conrsion{1..3,29} (4 alike) : DataTypeConversion  OutDataTypeStr=single
  Data Type Conrsion10 : DataTypeConversion  OutDataTypeStr=uint8
  Data Type Conrsion{4..8} (5 alike) : DataTypeConversion  OutDataTypeStr=boolean
  Data Type Conrsion9 : DataTypeConversion  OutDataTypeStr=uint8
  DriverRequest : Outport  VectorParamsAs1DForOutWhenUnconnected=off
  wires:
  Data Type Conrsion29/1 -> Bus Creator3/1
  Data Type Conrsion3/1 -> Bus Creator3/4
  Data Type Conrsion2/1 -> Bus Creator3/3
  Data Type Conrsion4/1 -> Bus Creator3/5
  Data Type Conrsion1/1 -> Bus Creator3/2
  Data Type Conrsion6/1 -> Bus Creator3/7
  Data Type Conrsion7/1 -> Bus Creator3/8
  Data Type Conrsion8/1 -> Bus Creator3/9
  Data Type Conrsion5/1 -> Bus Creator3/6
  Data Type Conrsion9/1 -> Bus Creator3/10
  Bus Creator3/1 -> DriverRequest/1  "DriverRequest"
  Constant8/1 -> Data Type Conrsion29/1
  Constant1/1 -> Data Type Conrsion1/1
  Constant2/1 -> Data Type Conrsion2/1
  Constant3/1 -> Data Type Conrsion3/1
  Constant4/1 -> Data Type Conrsion4/1
  Constant5/1 -> Data Type Conrsion5/1
  Constant6/1 -> Data Type Conrsion6/1
  Constant7/1 -> Data Type Conrsion7/1
  Constant9/1 -> Data Type Conrsion8/1
  Constant10/1 -> Data Type Conrsion9/1
  Constant11/1 -> Data Type Conrsion10/1
  Data Type Conrsion10/1 -> Bus Creator3/11

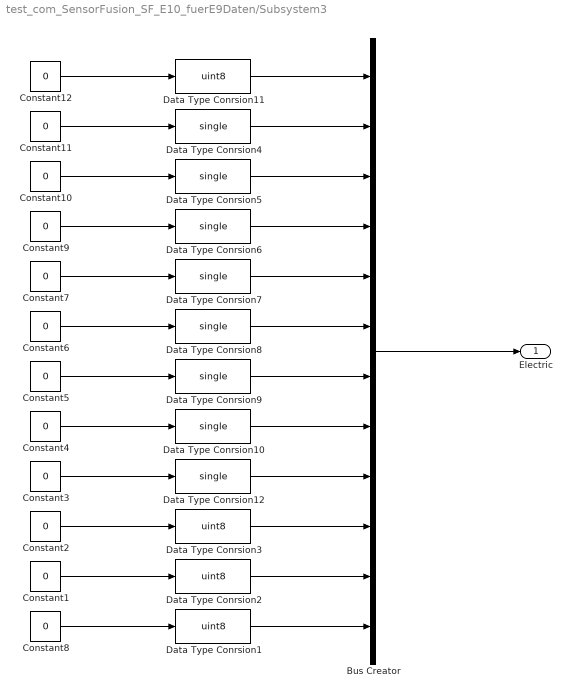
== system test_com_SensorFusion_SF_E10_fuerE9Daten/Subsystem3 ==
  Bus Creator : BusCreator  Inputs=12  OutDataTypeStr=Bus: control_Electric
      settings: InheritFromInputs=off
  Constant{1..12} (12 alike) : Constant  Value=0
  Data Type Conrsion{1..3,11} (4 alike) : DataTypeConversion  OutDataTypeStr=uint8
  Data Type Conrsion{4..10,12} (8 alike) : DataTypeConversion  OutDataTypeStr=single
  Electric : Outport  OutDataTypeStr=Bus: control_Electric  VectorParamsAs1DForOutWhenUnconnected=off
  wires:
  Bus Creator/1 -> Electric/1
  Constant8/1 -> Data Type Conrsion1/1
  Data Type Conrsion1/1 -> Bus Creator/12
  Data Type Conrsion2/1 -> Bus Creator/11
  Constant1/1 -> Data Type Conrsion2/1
  Constant2/1 -> Data Type Conrsion3/1
  Data Type Conrsion3/1 -> Bus Creator/10
  Constant3/1 -> Data Type Conrsion12/1
  Data Type Conrsion12/1 -> Bus Creator/9
  Constant4/1 -> Data Type Conrsion10/1
  Data Type Conrsion10/1 -> Bus Creator/8
  Constant5/1 -> Data Type Conrsion9/1
  Data Type Conrsion9/1 -> Bus Creator/7
  Constant6/1 -> Data Type Conrsion8/1
  Data Type Conrsion8/1 -> Bus Creator/6
  Constant7/1 -> Data Type Conrsion7/1
  Data Type Conrsion7/1 -> Bus Creator/5
  Constant9/1 -> Data Type Conrsion6/1
  Data Type Conrsion6/1 -> Bus Creator/4
  Constant10/1 -> Data Type Conrsion5/1
  Data Type Conrsion5/1 -> Bus Creator/3
  Constant11/1 -> Data Type Conrsion4/1
  Data Type Conrsion4/1 -> Bus Creator/2
  Constant12/1 -> Data Type Conrsion11/1
  Data Type Conrsion11/1 -> Bus Creator/1

== system test_com_SensorFusion_SF_E10_fuerE9Daten/Subsystem4 ==
  Constant8 : Constant  Value=0
  Data Type Conrsion29 : DataTypeConversion
  DriverDemand : Outport  VectorParamsAs1DForOutWhenUnconnected=off
  wires:
  Data Type Conrsion29/1 -> DriverDemand/1  "DriverDemand"
  Constant8/1 -> Data Type Conrsion29/1

== system test_com_SensorFusion_SF_E10_fuerE9Daten/Subsystem5 ==
  note: Wenn die Input-Daten Motordrehzahlen sind, dann sollte diese Konstatne 1 sein
      | Wenn die Input-Daten bereits Raddrehzahlen sind, dann sollte diese Konstante 2 sein
      |
      | if input-data are motor speeds than this constant should be 1
      | if input-data already are wheelspeeds than this constant should be 2
  " " : Inport
  In2 : Inport  Port=2
  In3 : Inport  Port=3
  In4 : Inport  Port=4
  Constant : Constant
  Gain1 : Gain  Gain=(60*gearbox_ratio)/(2*pi)
  Gain3 : Gain  Gain=(2*pi)/(60*gearbox_ratio)
  Multiport Switch : MultiPortSwitch  Inputs=2
  Multiport Switch1 : MultiPortSwitch  Inputs=2
  Mux : Mux
  wheelSpeed : Outport  VectorParamsAs1DForOutWhenUnconnected=off
  motorSpeed : Outport  Port=2  VectorParamsAs1DForOutWhenUnconnected=off
  wires:
  In3/1 -> Mux/3
  In4/1 -> Mux/4
  In2/1 -> Mux/2
  " "/1 -> Mux/1
  Mux/1 -> Multiport Switch/3, Gain1/1, Multiport Switch1/2, Gain3/1  "wheelSpeed"
  Gain3/1 -> Multiport Switch/2
  Gain1/1 -> Multiport Switch1/3
  Multiport Switch/1 -> wheelSpeed/1
  Multiport Switch1/1 -> motorSpeed/1
  Constant/1 -> Multiport Switch1/1, Multiport Switch/1

== system test_com_SensorFusion_SF_E10_fuerE9Daten/Subsystem6 ==
  Constant{,1..3} (4 alike) : Constant  Value=0
  Data Type Conrsion{19..22} (4 alike) : DataTypeConversion  OutDataTypeStr=single
  Mux : Mux
  wheelTorque : Outport  VectorParamsAs1DForOutWhenUnconnected=off
  wires:
  Constant2/1 -> Data Type Conrsion21/1
  Constant3/1 -> Data Type Conrsion22/1
  Constant/1 -> Data Type Conrsion19/1
  Constant1/1 -> Data Type Conrsion20/1
  Data Type Conrsion21/1 -> Mux/3
  Data Type Conrsion22/1 -> Mux/4
  Data Type Conrsion20/1 -> Mux/2
  Data Type Conrsion19/1 -> Mux/1
  Mux/1 -> wheelTorque/1  "wheelSpeed"

== system test_com_SensorFusion_SF_E10_fuerE9Daten/Subsystem7 ==
  Constant{,1..3} (4 alike) : Constant  Value=0
  Data Type Conrsion{19..22} (4 alike) : DataTypeConversion  OutDataTypeStr=single
  Mux : Mux
  motorTemp : Outport  VectorParamsAs1DForOutWhenUnconnected=off
  wires:
  Mux/1 -> motorTemp/1  "wheelSpeed"
  Data Type Conrsion19/1 -> Mux/1
  Data Type Conrsion20/1 -> Mux/2
  Data Type Conrsion22/1 -> Mux/4
  Data Type Conrsion21/1 -> Mux/3
  Constant1/1 -> Data Type Conrsion20/1
  Constant/1 -> Data Type Conrsion19/1
  Constant3/1 -> Data Type Conrsion22/1
  Constant2/1 -> Data Type Conrsion21/1

== system test_com_SensorFusion_SF_E10_fuerE9Daten/Subsystem8 ==
  Constant{,1..3} (4 alike) : Constant  Value=0
  Data Type Conrsion{19..22} (4 alike) : DataTypeConversion  OutDataTypeStr=single
  Mux : Mux
  inverterTemp : Outport  VectorParamsAs1DForOutWhenUnconnected=off
  wires:
  Constant2/1 -> Data Type Conrsion21/1
  Constant3/1 -> Data Type Conrsion22/1
  Constant/1 -> Data Type Conrsion19/1
  Constant1/1 -> Data Type Conrsion20/1
  Data Type Conrsion21/1 -> Mux/3
  Data Type Conrsion22/1 -> Mux/4
  Data Type Conrsion20/1 -> Mux/2
  Data Type Conrsion19/1 -> Mux/1
  Mux/1 -> inverterTemp/1  "wheelSpeed"

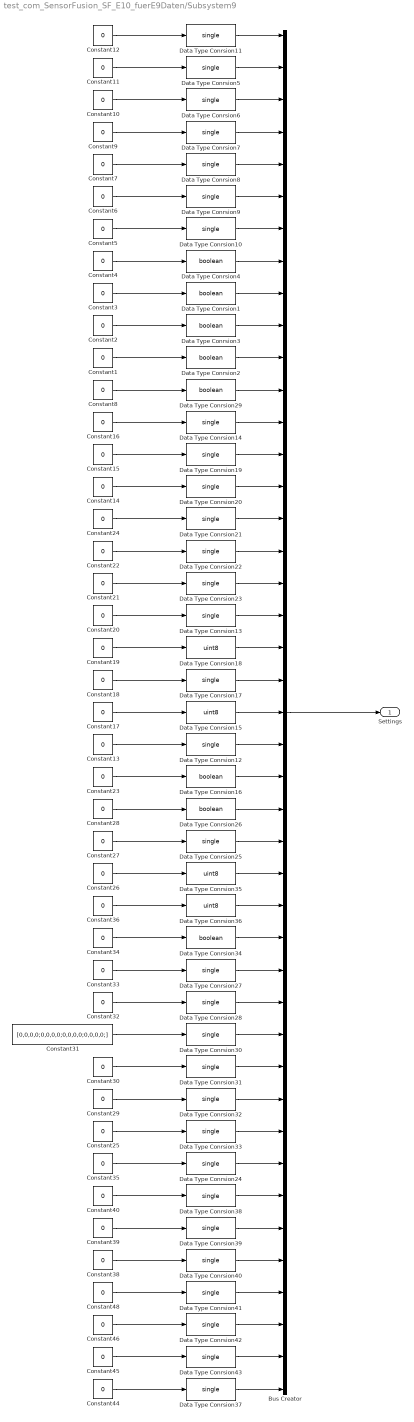
== system test_com_SensorFusion_SF_E10_fuerE9Daten/Subsystem9 ==
  Bus Creator : BusCreator  Inputs=43
  Constant{1..30,32..36,38..40,44..46,48} (42 alike) : Constant  Value=0
  Constant31 : Constant  Value=[0,0,0,0;0,0,0,0;0,0,0,0;0,0,0,0;]
  Data Type Conrsion{1..4,16,26,29,34} (8 alike) : DataTypeConversion  OutDataTypeStr=boolean
  Data Type Conrsion{5..14,17,19..25,27..28,30..33,37..43} (31 alike) : DataTypeConversion  OutDataTypeStr=single
  Data Type Conrsion{15,18,35..36} (4 alike) : DataTypeConversion  OutDataTypeStr=uint8
  Settings : Outport  VectorParamsAs1DForOutWhenUnconnected=off
  wires:
  Constant12/1 -> Data Type Conrsion11/1
  Constant11/1 -> Data Type Conrsion5/1
  Constant10/1 -> Data Type Conrsion6/1
  Constant9/1 -> Data Type Conrsion7/1
  Constant7/1 -> Data Type Conrsion8/1
  Constant6/1 -> Data Type Conrsion9/1
  Constant5/1 -> Data Type Conrsion10/1
  Constant4/1 -> Data Type Conrsion4/1
  Constant3/1 -> Data Type Conrsion1/1
  Constant2/1 -> Data Type Conrsion3/1
  Constant1/1 -> Data Type Conrsion2/1
  Constant8/1 -> Data Type Conrsion29/1
  Bus Creator/1 -> Settings/1
  Constant23/1 -> Data Type Conrsion16/1
  Constant13/1 -> Data Type Conrsion12/1
  Constant17/1 -> Data Type Conrsion15/1
  Constant18/1 -> Data Type Conrsion17/1
  Constant19/1 -> Data Type Conrsion18/1
  Constant20/1 -> Data Type Conrsion13/1
  Constant21/1 -> Data Type Conrsion23/1
  Constant22/1 -> Data Type Conrsion22/1
  Constant24/1 -> Data Type Conrsion21/1
  Constant14/1 -> Data Type Conrsion20/1
  Constant15/1 -> Data Type Conrsion19/1
  Constant16/1 -> Data Type Conrsion14/1
  Constant28/1 -> Data Type Conrsion26/1
  Constant27/1 -> Data Type Conrsion25/1
  Constant26/1 -> Data Type Conrsion35/1
  Constant36/1 -> Data Type Conrsion36/1
  Constant34/1 -> Data Type Conrsion34/1
  Constant33/1 -> Data Type Conrsion27/1
  Constant32/1 -> Data Type Conrsion28/1
  Constant31/1 -> Data Type Conrsion30/1
  Constant30/1 -> Data Type Conrsion31/1
  Constant29/1 -> Data Type Conrsion32/1
  Constant25/1 -> Data Type Conrsion33/1
  Constant35/1 -> Data Type Conrsion24/1
  Constant44/1 -> Data Type Conrsion37/1
  Constant45/1 -> Data Type Conrsion43/1
  Constant46/1 -> Data Type Conrsion42/1
  Constant48/1 -> Data Type Conrsion41/1
  Constant38/1 -> Data Type Conrsion40/1
  Constant39/1 -> Data Type Conrsion39/1
  Constant40/1 -> Data Type Conrsion38/1
  Data Type Conrsion37/1 -> Bus Creator/43
  Data Type Conrsion43/1 -> Bus Creator/42
  Data Type Conrsion42/1 -> Bus Creator/41
  Data Type Conrsion41/1 -> Bus Creator/40
  Data Type Conrsion40/1 -> Bus Creator/39
  Data Type Conrsion39/1 -> Bus Creator/38
  Data Type Conrsion38/1 -> Bus Creator/37
  Data Type Conrsion24/1 -> Bus Creator/36
  Data Type Conrsion33/1 -> Bus Creator/35
  Data Type Conrsion32/1 -> Bus Creator/34
  Data Type Conrsion31/1 -> Bus Creator/33
  Data Type Conrsion30/1 -> Bus Creator/32
  Data Type Conrsion28/1 -> Bus Creator/31
  Data Type Conrsion27/1 -> Bus Creator/30
  Data Type Conrsion34/1 -> Bus Creator/29
  Data Type Conrsion36/1 -> Bus Creator/28
  Data Type Conrsion35/1 -> Bus Creator/27
  Data Type Conrsion25/1 -> Bus Creator/26
  Data Type Conrsion26/1 -> Bus Creator/25
  Data Type Conrsion16/1 -> Bus Creator/24
  Data Type Conrsion12/1 -> Bus Creator/23
  Data Type Conrsion15/1 -> Bus Creator/22
  Data Type Conrsion17/1 -> Bus Creator/21
  Data Type Conrsion18/1 -> Bus Creator/20
  Data Type Conrsion13/1 -> Bus Creator/19
  Data Type Conrsion23/1 -> Bus Creator/18
  Data Type Conrsion22/1 -> Bus Creator/17
  Data Type Conrsion21/1 -> Bus Creator/16
  Data Type Conrsion20/1 -> Bus Creator/15
  Data Type Conrsion19/1 -> Bus Creator/14
  Data Type Conrsion14/1 -> Bus Creator/13
  Data Type Conrsion29/1 -> Bus Creator/12
  Data Type Conrsion2/1 -> Bus Creator/11
  Data Type Conrsion3/1 -> Bus Creator/10
  Data Type Conrsion1/1 -> Bus Creator/9
  Data Type Conrsion4/1 -> Bus Creator/8
  Data Type Conrsion10/1 -> Bus Creator/7
  Data Type Conrsion9/1 -> Bus Creator/6
  Data Type Conrsion8/1 -> Bus Creator/5
  Data Type Conrsion7/1 -> Bus Creator/4
  Data Type Conrsion6/1 -> Bus Creator/3
  Data Type Conrsion5/1 -> Bus Creator/2
  Data Type Conrsion11/1 -> Bus Creator/1

== system test_com_SensorFusion_SF_E10_fuerE9Daten/0213_PlausibiltyCheck1/9DFront_Plausibility ==
  In : Inport  OutDataTypeStr=Bus: control_9D
  Bus Creator : BusCreator  Inputs=16  OutDataTypeStr=Bus: control_9D
  Bus Selector : BusSelector  OutputSignals=AccX,AccX_Sq,AccY,AccY_Sq,AccZ,AccZ_Sq,RollRate,RollRate_Sq,PitchRate,PitchRate_Sq,YawRate,YawRate_Sq,MagX,MagY,MagZ,Temperature
  Plausibility_Test_AccX : SignalProcessingSensorFusionLib/Plausibility_AllTests  alpha=0.3  checkGradient=off  deviation=0  threshold=0  alpha2=0  increasingPercentage=0  signalBounds=1e-8  stepDelay=25  upperBound=50  lowerBound=-50  useAlternativeValue=off  useManualAlternativeValue=off  manualAlternativeValue=0
  Plausibility_Test_AccY : SignalProcessingSensorFusionLib/Plausibility_AllTests  alpha=0.3  checkGradient=off  deviation=0  threshold=0  alpha2=0  increasingPercentage=0  signalBounds=1e-8  stepDelay=25  upperBound=50  lowerBound=-50  useAlternativeValue=off  useManualAlternativeValue=off  manualAlternativeValue=0
  Plausibility_Test_AccZ : SignalProcessingSensorFusionLib/Plausibility_AllTests  alpha=0.3  checkGradient=off  deviation=0  threshold=0  alpha2=0  increasingPercentage=0  signalBounds=1e-8  stepDelay=25  upperBound=50  lowerBound=-50  useAlternativeValue=off  useManualAlternativeValue=off  manualAlternativeValue=0
  Plausibility_Test_PitchRate : SignalProcessingSensorFusionLib/Plausibility_AllTests  alpha=0.3  checkGradient=off  deviation=0  threshold=0  alpha2=0  increasingPercentage=0  signalBounds=1e-8  stepDelay=25  upperBound=1.6  lowerBound=-1.6  useAlternativeValue=off  useManualAlternativeValue=off  manualAlternativeValue=0
  Plausibility_Test_RollRate : SignalProcessingSensorFusionLib/Plausibility_AllTests  alpha=0.3  checkGradient=off  deviation=0  threshold=0  alpha2=0  increasingPercentage=0  signalBounds=1e-8  stepDelay=25  upperBound=1.6  lowerBound=-1.6  useAlternativeValue=off  useManualAlternativeValue=off  manualAlternativeValue=0
  Plausibility_Test_YawRate : SignalProcessingSensorFusionLib/Plausibility_AllTests  alpha=0.3  checkGradient=off  deviation=0  threshold=0  alpha2=0  increasingPercentage=0  signalBounds=1e-8  stepDelay=25  upperBound=3  lowerBound=-3  useAlternativeValue=off  useManualAlternativeValue=off  manualAlternativeValue=0
  Out : Outport  VectorParamsAs1DForOutWhenUnconnected=off
  wires:
  Plausibility_Test_AccY/2 -> Bus Creator/12  "AccY_Sq"
  Plausibility_Test_AccY/1 -> Bus Creator/2  "AccY"
  Bus Selector/2 -> Plausibility_Test_AccX/2  "<AccX_Sq>"
  Bus Selector/4 -> Plausibility_Test_AccY/2  "<AccY_Sq>"
  Bus Selector/3 -> Plausibility_Test_AccY/1  "<AccY>"
  In/1 -> Bus Selector/1
  Plausibility_Test_AccX/1 -> Bus Creator/1  "AccX"
  Bus Selector/1 -> Plausibility_Test_AccX/1  "<AccX>"
  Plausibility_Test_AccX/2 -> Bus Creator/11  "AccX_Sq"
  Bus Selector/6 -> Plausibility_Test_AccZ/2  "<AccZ_Sq>"
  Plausibility_Test_AccZ/1 -> Bus Creator/3  "AccZ"
  Bus Selector/5 -> Plausibility_Test_AccZ/1  "<AccZ>"
  Bus Selector/8 -> Plausibility_Test_RollRate/2  "<RollRate_Sq>"
  Bus Selector/7 -> Plausibility_Test_RollRate/1  "<RollRate>"
  Plausibility_Test_RollRate/1 -> Bus Creator/4  "RollRate"
  Bus Creator/1 -> Out/1
  Bus Selector/10 -> Plausibility_Test_PitchRate/2  "<PitchRate_Sq>"
  Plausibility_Test_PitchRate/1 -> Bus Creator/5  "PitchRate"
  Bus Selector/12 -> Plausibility_Test_YawRate/2  "<YawRate_Sq>"
  Plausibility_Test_YawRate/1 -> Bus Creator/6  "YawRate"
  Bus Selector/9 -> Plausibility_Test_PitchRate/1  "<PitchRate>"
  Bus Selector/11 -> Plausibility_Test_YawRate/1  "<YawRate>"
  Plausibility_Test_YawRate/2 -> Bus Creator/16  "YawRate_Sq"
  Plausibility_Test_PitchRate/2 -> Bus Creator/15  "PitchRate_Sq"
  Plausibility_Test_RollRate/2 -> Bus Creator/14  "RollRate_Sq"
  Plausibility_Test_AccZ/2 -> Bus Creator/13  "AccZ_Sq"
  Bus Selector/13 -> Bus Creator/7  "<MagX>"
  Bus Selector/14 -> Bus Creator/8  "<MagY>"
  Bus Selector/15 -> Bus Creator/9  "<MagZ>"
  Bus Selector/16 -> Bus Creator/10  "<Temperature>"
